simulink model "example_Storage_type2conf"  (R2016b)
settings: Solver=ode45  StartTime=0.0  StopTime=3*3600-2  MaxStep=300  RelTol=1e-3  EnableMultiTasking=on
undefined symbols (not defined in the file): path_carnot
libraries: carnot x14, simulink x3
settings Model: Creator=drhf  LastModifiedBy=drhf
settings DataIOCC: LimitDataPoints=on  SaveFormat=Array
settings OptimizationCC: ExpressionDepthLimit=2147483647  LifeSpan=inf
settings DebuggingCC: UnderspecifiedInitializationDetection=Classic  MergeDetectMultiDrivingBlocksExec=none  SolverPrmCheckMsg=warning  StateNameClashWarn=warning  SFUnexpectedBacktrackingDiag=warning  SFNoUnconditionalDefaultTransitionDiag=warning  SFExecutionAtInitializationDiag=none
settings HardwareCC: ProdBitPerPointer=32  ProdBitPerSizeT=32  ProdBitPerPtrDiffT=32  ProdLargestAtomicFloat=None  ProdIntDivRoundTo=Undefined  ProdEndianess=Unspecified  ProdWordSize=32  ProdHWDeviceType=32-bit Generic
settings ModelReferenceCC: PropagateSignalLabelsOutOfModel=off
settings GRTTargetCC: TargetLangStandard=C89/C90 (ANSI)  GeneratePreprocessorConditionals=Disable all  CombineOutputUpdateFcns=off  GRTInterface=on
settings ConfigComp: CovMetricSettings=dw  CovHtmlReporting=on  CovSaveCumulativeToWorkspaceVar=on  CovSaveSingleToWorkspaceVar=on  CovExternalEMLEnable=off

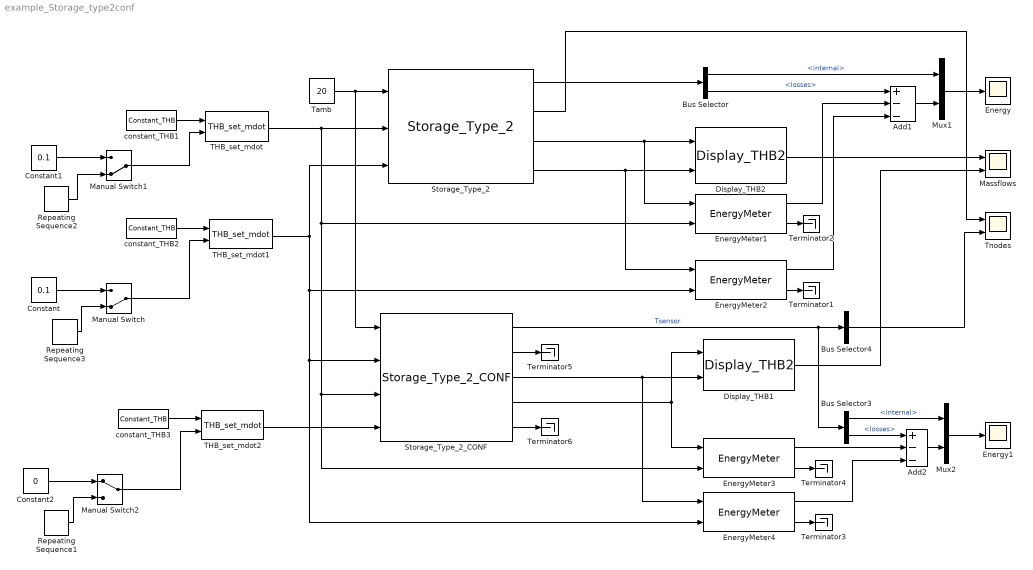
== system example_Storage_type2conf ==
  Add1 : Sum  Inputs=+--
  Add2 : Sum  Inputs=+--
  Bus Selector : BusSelector  OutputSignals=energy.internal,energy.losses
  Bus Selector3 : BusSelector  OutputSignals=energy.internal,energy.losses
  Bus Selector4 : BusSelector  OutputSignals=Tnodes  OutputAsBus=on
  Constant : Constant  Value=0.1
  Constant1 : Constant  Value=0.1
  Constant2 : Constant  Value=0
  Display_THB1 : carnot/Outputs/Display_THB2  t=off  m=on  p=off  id=off  mix=off  d=off
  Display_THB2 : carnot/Outputs/Display_THB2  t=off  m=on  p=off  id=off  mix=off  d=off
  Energy : Scope
  Energy1 : Scope
  EnergyMeter{1..4} (4 alike) : carnot/Control/EnergyMeter
  Manual Switch : ManualSwitch  CurrentSetting=0
  Manual Switch1 : ManualSwitch  CurrentSetting=0
  Manual Switch2 : ManualSwitch
  Massflows : Scope  NumInputPorts=2
  Mux1 : Mux  Inputs=2
  Mux2 : Mux  Inputs=2
  Repeating Sequence1 : simulink/Sources/Repeating Sequence  rep_seq_t=[0 1 1.01 2 2.01 3]*3600  rep_seq_y=[0 0 0.01 0.01 0 0]
  Repeating Sequence2 : simulink/Sources/Repeating Sequence  rep_seq_t=[0 1 1.01 2 2.01 2.9 2.91 3.1]*3600  rep_seq_y=[0.12 0.12 0.15 0.15 0.1 0.1 0 0]
  Repeating Sequence3 : simulink/Sources/Repeating Sequence  rep_seq_t=[0 1 1.01 2 2.01 3]*3600  rep_seq_y=[0.12 0.12 0.1 0.1 0.15 0.15]
  Storage_Type_2 : carnot/Storage/Thermal/Storage_Type_2  uloss=1  ubot=1  utop=1  cond=1  volume=0.3  dia=0.5  pos=standing cylinder  h_in_chg=0.5  h_out_chg=0.1  ua0=80  uam=0.2  uat=0.5  dplin_chg=100  dpqua_chg=100  h_in=0  h_out=1  pipedia=0.03  t0=[10:5:55]  nodes=10  mpoints=10
  Storage_Type_2_CONF : carnot/Storage/Thermal/Storage_Type_2_CONF  t0=[10:5:55]  hgt=1.5279  stgtype=2  tini=[10 15 20 25 30 35 40 45 50 55]  mpts=[1 2 3 4 5 6 7 8 9 10]  PathName=fullfile(path_carnot('libsl'),'Storage','Thermal','Storage_Type_2_CONF','parameter_set')  FileName='StorageType2_300_L.mat'  userPath=off  userParam=off  uwall=1  ubot=1  utop=1  axcond=1  volume=0.3  dia=0.5  standing=standing cylinder  nodes=10  mpoints=10  Tsensor=0.5  hx1inlet=0.45  hx1outlet=0  hx1dia=0.03  hx1uac=50  hx1uam=0.15  hx1uat=0.6  hx1dpqua=20  hx1dplin=20  pipe1inlet=0  pipe1outlet=1  pipe1dia=0.03  pipe2inlet=0.6  pipe2outlet=1  pipe2dia=0.03
  THB_set_mdot : carnot/Source/Simple/THB_set_mdot
  THB_set_mdot1 : carnot/Source/Simple/THB_set_mdot
  THB_set_mdot2 : carnot/Source/Simple/THB_set_mdot
  Tamb : Constant  Value=20
  Terminator{1..6} (6 alike) : Terminator
  Tnodes : Scope  NumInputPorts=2
  constant_THB1 : carnot/Source/Simple/Constant_THB  t=55  mdot=0*100/3600  p=1e5  mID=Full Pressure Drop with Static Height  fluid=Water  mix=0  mix2=0  mix3=0  dia=0.02  hgt=0
  constant_THB2 : carnot/Source/Simple/Constant_THB  t=10  mdot=100/3600  p=1e5  mID=Full Pressure Drop with Static Height  fluid=Water  mix=0  mix2=0  mix3=0  dia=0.02  hgt=0
  constant_THB3 : carnot/Source/Simple/Constant_THB  t=55  mdot=0  p=1e5  mID=Full Pressure Drop with Static Height  fluid=Water  mix=0  mix2=0  mix3=0  dia=0.02  hgt=0
  wires:
  Bus Selector/1 -> Mux1/1  "<internal>"
  Tamb/1 -> Storage_Type_2_CONF/1, Storage_Type_2/1
  THB_set_mdot/1 -> Storage_Type_2_CONF/3, EnergyMeter3/2, EnergyMeter1/2, Storage_Type_2/2
  THB_set_mdot1/1 -> Storage_Type_2/3, EnergyMeter2/2, Storage_Type_2_CONF/2, EnergyMeter4/2
  Storage_Type_2/1 -> Bus Selector/1
  Storage_Type_2/2 -> Tnodes/1
  Storage_Type_2/3 -> Display_THB2/1, EnergyMeter1/1
  Storage_Type_2/4 -> EnergyMeter2/1, Display_THB2/2
  Mux1/1 -> Energy/1
  EnergyMeter2/2 -> Terminator1/1
  constant_THB1/1 -> THB_set_mdot/1
  constant_THB2/1 -> THB_set_mdot1/1
  Manual Switch1/1 -> THB_set_mdot/2
  Manual Switch/1 -> THB_set_mdot1/2
  Constant/1 -> Manual Switch/1
  Repeating Sequence3/1 -> Manual Switch/2
  Constant1/1 -> Manual Switch1/1
  Repeating Sequence2/1 -> Manual Switch1/2
  EnergyMeter1/2 -> Terminator2/1
  EnergyMeter2/1 -> Add1/3
  EnergyMeter1/1 -> Add1/2
  Storage_Type_2_CONF/1 -> Bus Selector3/1, Bus Selector4/1  "Tsensor"
  Mux2/1 -> Energy1/1
  Storage_Type_2_CONF/4 -> Display_THB1/1, EnergyMeter3/1
  Add1/1 -> Mux1/2
  EnergyMeter3/1 -> Add2/2
  EnergyMeter4/1 -> Add2/3
  Add2/1 -> Mux2/2
  Storage_Type_2_CONF/3 -> EnergyMeter4/1, Display_THB1/2
  EnergyMeter4/2 -> Terminator3/1
  EnergyMeter3/2 -> Terminator4/1
  Display_THB2/1 -> Massflows/1
  Display_THB1/1 -> Massflows/2
  constant_THB3/1 -> THB_set_mdot2/1
  Manual Switch2/1 -> THB_set_mdot2/2
  Constant2/1 -> Manual Switch2/1
  Repeating Sequence1/1 -> Manual Switch2/2
  THB_set_mdot2/1 -> Storage_Type_2_CONF/4
  Bus Selector4/1 -> Tnodes/2
  Storage_Type_2_CONF/2 -> Terminator5/1
  Storage_Type_2_CONF/5 -> Terminator6/1
  Bus Selector3/1 -> Mux2/1  "<internal>"
  Bus Selector/2 -> Add1/1  "<losses>"
  Bus Selector3/2 -> Add2/1  "<losses>"
